simulink model "ZeroLagGuidance"  (R2020b)
settings: Solver=ode4  StartTime=0.0  StopTime=10.0  FixedStep=h  RelTol=1e-3
undefined symbols (not defined in the file): N_prime, nt, Tf, Vc, y, yDot
settings Model: Creator=dariusmensah  LastModifiedBy=dariusmensah

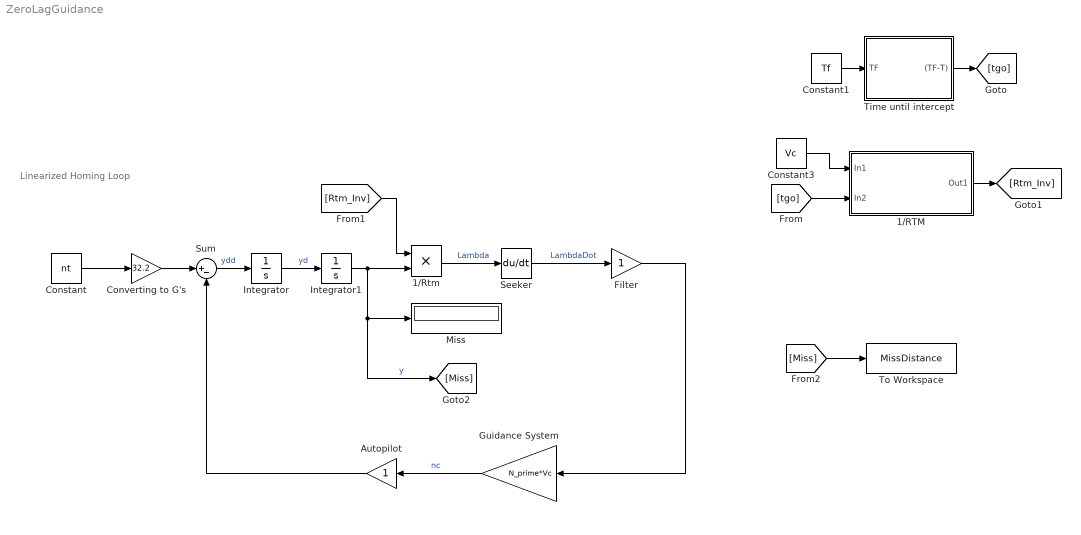
== system ZeroLagGuidance ==
  note: Linearized Homing Loop
  1/RTM : Subsystem
  1/Rtm : Product
  Autopilot : Gain
  Constant : Constant  Value=nt
  Constant1 : Constant  Value=Tf
  Constant3 : Constant  Value=Vc
  Converting to G's : Gain  Gain=32.2
  Filter : Gain
  Guidance System : Gain  Gain=N_prime*Vc
  Integrator : Integrator  InitialCondition=yDot
  Integrator1 : Integrator  InitialCondition=y
  Miss : Display
  Seeker : Derivative
  Sum : Sum  Inputs=|+-
  Time until intercept : Subsystem
  To Workspace : ToWorkspace  VariableName=MissDistance  SaveFormat=Structure With Time  SampleTime=-1
  wires:
  Sum/1 -> Integrator/1  "ydd"
  Integrator/1 -> Integrator1/1  "yd"
  Integrator1/1 -> [Miss], Miss/1, 1/Rtm/2  "y"
  1/Rtm/1 -> Seeker/1  "Lambda"
  Seeker/1 -> Filter/1  "LambdaDot"
  Filter/1 -> Guidance System/1
  Guidance System/1 -> Autopilot/1  "nc"
  Autopilot/1 -> Sum/2
  Constant1/1 -> Time until intercept/1(TF)
  Time until intercept/1((TF-T)) -> [tgo]
  Constant3/1 -> 1/RTM/1(In1)
  [tgo] -> 1/RTM/2(In2)
  1/RTM/1(Out1) -> [Rtm_Inv]
  [Rtm_Inv] -> 1/Rtm/1
  [Miss] -> To Workspace/1
  Converting to G's/1 -> Sum/1
  Constant/1 -> Converting to G's/1

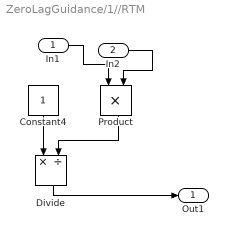
== system ZeroLagGuidance/1//RTM ==
  In1 : Inport
  In2 : Inport  Port=2
  Constant4 : Constant
  Divide : Product  Inputs=*/
  Product : Product
  Out1 : Outport
  wires:
  In1/1 -> Product/1
  In2/1 -> Product/2
  Constant4/1 -> Divide/1
  Divide/1 -> Out1/1
  Product/1 -> Divide/2

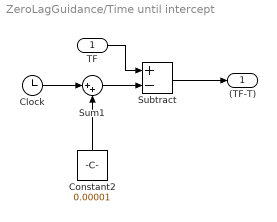
== system ZeroLagGuidance/Time until intercept ==
  TF : Inport
  Clock : Clock
  Constant2 : Constant  Value=0.00001
  Subtract : Sum  Inputs=+-
  Sum1 : Sum  Inputs=|++
  (TF-T) : Outport
  wires:
  TF/1 -> Subtract/1
  Subtract/1 -> (TF-T)/1
  Sum1/1 -> Subtract/2
  Clock/1 -> Sum1/1
  Constant2/1 -> Sum1/2
